simulink model "SPWM"  (R2018b)
settings: Solver=FixedStepAuto  StartTime=0.0  StopTime=0.02  RelTol=1e-3
undefined symbols (not defined in the file): gcbh, Newton, Raphson, sps_rtmsupport
libraries: powerlib x60, powerlib_meascontrol x21, simulink x14, dspstat3 x1
(part 1 of 2)
settings Model: Creator=Lenovo  LastModifiedBy=Lenovo

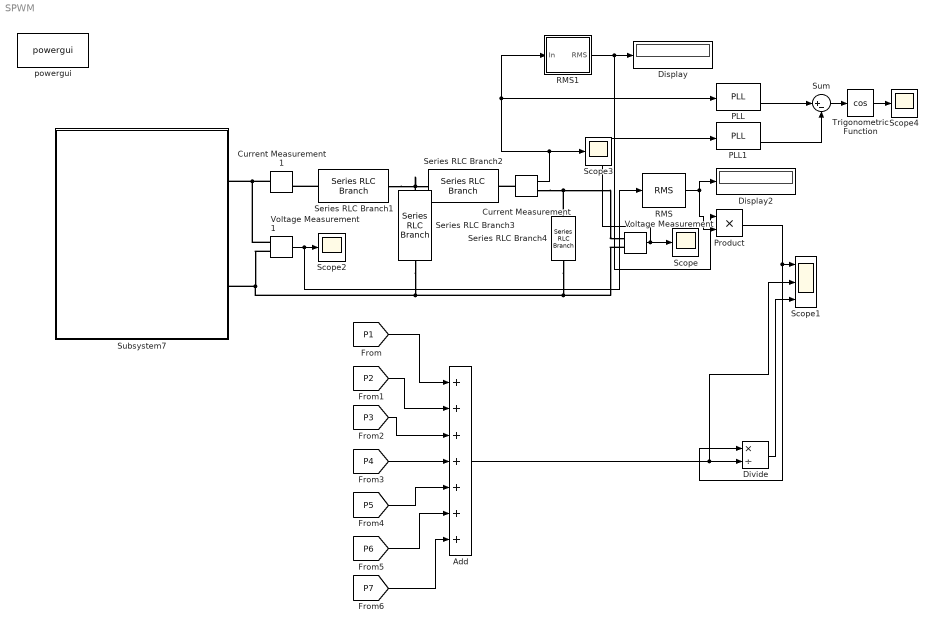
== system SPWM ==
  Add : Sum  Inputs=+++++++
  Current Measurement : powerlib/Measurements/Current Measurement  PhasorSimulation=off  OutputType=Complex  PSBequivalent=0
  Current Measurement1 : powerlib/Measurements/Current Measurement  PhasorSimulation=off  OutputType=Complex  PSBequivalent=0
  Display : Display
  Display2 : Display
  Divide : Product  Inputs=*/
  PLL : powerlib_meascontrol/PLL/PLL  Fmin=45  Par_Init=[0, 50]  ParK=[180, 3200, 1]  TcD=1e-4  MaxRateChangeFreq=12  FilterCutOffFreq=25  Ts=0  AGC=on
      settings: SourceProductName=Simscape Power Systems  SourceProductBaseCode=PS
  PLL1 : powerlib_meascontrol/PLL/PLL  Fmin=45  Par_Init=[0, 50]  ParK=[180, 3200, 1]  TcD=1e-4  MaxRateChangeFreq=12  FilterCutOffFreq=25  Ts=0  AGC=on
      settings: SourceProductName=Simscape Power Systems  SourceProductBaseCode=PS
  Product : Product
  RMS : powerlib_meascontrol/Measurements/RMS  TrueRMS=on  Freq=50  RMSInit=0  Ts=0
  RMS1 : Subsystem  DialogController=POWERSYS.PowerSysDialog  LoadFcn=sps_rtmsupport('LoadFcn', gcbh);  StartFcn=sps_rtmsupport('StartFcn', gcbh);  StopFcn=sps_rtmsupport('StopFcn', gcbh);  mask(RMS){TrueRMS=on, Freq=50, RMSInit=0, Ts=0}
      mask prompts: TrueRMS "True RMS value"; Freq "Fundamental frequency (Hz):"; RMSInit "Initial RMS value:"; Ts "Sample time:"
      mask help:
      | Measure the true root mean square (RMS) value of the input signal at the specified fundamental frequency.
      |
      | When True RMS value parameter is unchecked, the block outputs the RMS value of the fundamental component of the input signal.
      mask init:
      | [sps] = powericon('RMSInit',gcb,Freq,RMSInit,TrueRMS,Ts);
      settings: CopyFcn=sps_rtmsupport('CopyFcn', gcbh);  DeleteFcn=sps_rtmsupport('DeleteFcn', gcbh);  UndoDeleteFcn=sps_rtmsupport('UndoDeleteFcn', gcbh);  ModelCloseFcn=sps_rtmsupport('ModelCloseFcn', gcbh);  PreSaveFcn=sps_rtmsupport('PreSaveFcn', gcbh);  PostSaveFcn=sps_rtmsupport('PostSaveFcn', gcbh);  NameChangeFcn=sps_rtmsupport('NameChangeFcn', gcbh);  PreCopyFcn=sps_rtmsupport('PreCopyFcn', gcbh);  OpenFcn=sps_rtmsupport('OpenFcn', gcbh, [1]);  CloseFcn=sps_rtmsupport('CloseFcn', gcbh);  PreDeleteFcn=sps_rtmsupport('PreDeleteFcn', gcbh);
      mask Help: helpview(psbhelp);
      mask Display: color('blue');disp('RMS')
  Scope{,2..4} (4 alike) : Scope
  Scope1 : Scope  NumInputPorts=3
  Series RLC Branch1 : powerlib/Elements/Series RLC Branch  LConnTagsString=__new0  RConnTagsString=__new0  BranchType=L  Resistance=0.5  Inductance=0.32e-3  SetiL0=off  InitialCurrent=0  Capacitance=1e-6  Setx0=off  InitialVoltage=0  Measurements=None
  Series RLC Branch2 : powerlib/Elements/Series RLC Branch  LConnTagsString=__new0  RConnTagsString=__new0  BranchType=L  Resistance=0.5  Inductance=0.32e-3  SetiL0=off  InitialCurrent=0  Capacitance=1e-6  Setx0=off  InitialVoltage=0  Measurements=None
  Series RLC Branch3 : powerlib/Elements/Series RLC Branch  LConnTagsString=__new0  RConnTagsString=__new0  BranchType=C  Resistance=1  Inductance=1e-3  SetiL0=off  InitialCurrent=0  Capacitance=25e-4  Setx0=off  InitialVoltage=0  Measurements=None
  Series RLC Branch4 : powerlib/Elements/Series RLC Branch  LConnTagsString=__new0  RConnTagsString=__new0  BranchType=RL  Resistance=50  Inductance=50e-6  SetiL0=off  InitialCurrent=0  Capacitance=1e-6  Setx0=off  InitialVoltage=0  Measurements=None
  Subsystem7 : Subsystem
  Sum : Sum  Inputs=|+-
  Trigonometric Function : Trigonometry  Operator=cos
  Voltage Measurement : powerlib/Measurements/Voltage Measurement  PhasorSimulation=off  OutputType=Complex  PSBequivalent=0
  Voltage Measurement1 : powerlib/Measurements/Voltage Measurement  PhasorSimulation=off  OutputType=Complex  PSBequivalent=0
  powergui : powerlib/powergui  Priority=1  SimulationMode=Discrete  SampleTime=50e-6  frequency=60  Iterations=50  frequencyindice=0  Pbase=100e6  ErrMax=1e-4  UnitsV=kV  UnitsW=MW  buscounter=0  FunctionMessages=off  echomessages=off  EnableUseOfTLC=off  CurrentSourceSwitches=off  DisableSnubberDevices=off  DisableRonSwitches=off  DisableVfSwitches=off  DisplayEquations=off  SolverType=Tustin/Backward Euler (TBE)  Interpol=off  ExternalGateDelay=off  methode=off  Ts=100  x0status=blocks  SPID=off  SwTol=0  HookPort=off  RestoreLinks=warning  ResistiveCurrentMeasurement=off  Frange=[0:2:500]  Ylog=off  Xlog=on  ShowGrid=off  save=off  variable=ZData  structure=vinay3  ZoomFFT=off  StartTime=0.04  cycles=1  DisplayStyle=1  fundamental=50  FreqAxis=off  MaxFrequency=1000  frequencyindicesteady=1  RmsSteady=1  display=off
  wires:
  Voltage Measurement/1 -> PLL1/1, Scope/1
  Current Measurement/1 -> Scope3/1, RMS1/1(In), PLL/1
  Voltage Measurement1/1 -> RMS/1, Scope2/1
  RMS/1 -> Display2/1, Product/2
  [P1] -> Add/1
  [P2] -> Add/2
  [P3] -> Add/3
  [P4] -> Add/4
  [P5] -> Add/5
  [P6] -> Add/6
  [P7] -> Add/7
  Divide/1 -> Scope1/3
  RMS1/1(RMS) -> Product/1, Display/1
  Product/1 -> Divide/1, Scope1/1
  PLL/2 -> Sum/1
  PLL1/2 -> Sum/2
  Sum/1 -> Trigonometric Function/1
  Trigonometric Function/1 -> Scope4/1
  Add/1 -> Scope1/2, Divide/2
  connections:
  Subsystem7/RConn2 -- Series RLC Branch4/RConn1 -- Voltage Measurement/LConn2 -- Series RLC Branch3/RConn1 -- Voltage Measurement1/LConn2
  Series RLC Branch3/LConn1 -- Series RLC Branch1/RConn1 -- Series RLC Branch2/LConn1
  Voltage Measurement1/LConn1 -- Current Measurement1/LConn1 -- Subsystem7/RConn1
  Current Measurement/LConn1 -- Series RLC Branch2/RConn1
  Voltage Measurement/LConn1 -- Current Measurement/RConn1 -- Series RLC Branch4/LConn1
  Series RLC Branch1/LConn1 -- Current Measurement1/RConn1

== system SPWM/RMS1 ==
  In : Inport  SampleTime=Ts
  Constant : Constant  Value=TrueRMS
  Data Type Conversion : DataTypeConversion  OutDataTypeStr=boolean
  Logical Operator : Logic  Operator=NOT  AllPortsSameDT=off  OutDataTypeStr=boolean
  "RMS " : Subsystem
  Switch : Switch  Criteria=u2 ~= 0  Threshold=0.5
  "TrueRMS " : Subsystem
  RMS : Outport  SampleTime=Ts
  tag scope: Iooooobvw=global
  wires:
  In/1 -> "TrueRMS "/1(In), "RMS "/1(In)
  Switch/1 -> [Iooooobvw], RMS/1
  "TrueRMS "/1(RMS) -> Switch/1
  "RMS "/1(RMS) -> Switch/3
  Constant/1 -> Data Type Conversion/1
  Data Type Conversion/1 -> Logical Operator/1, "TrueRMS "/Enable, Switch/2
  Logical Operator/1 -> "RMS "/Enable

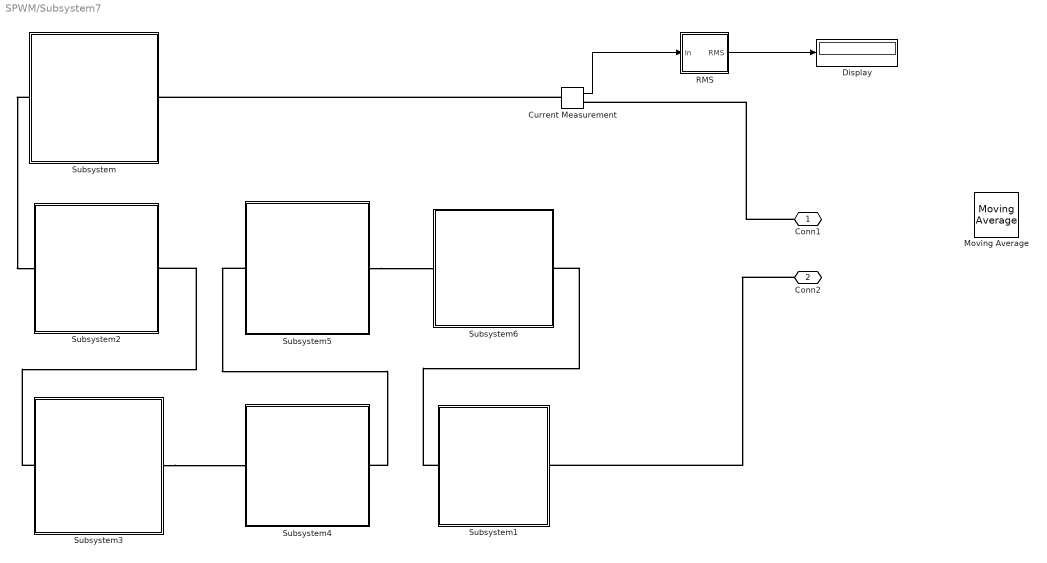
== system SPWM/Subsystem7 ==
  Current Measurement : powerlib/Measurements/Current Measurement  PhasorSimulation=off  OutputType=Complex  PSBequivalent=0
  Display : Display
  Moving Average : dspstat3/Moving Average  Method=Sliding window  ForgettingFactorPort=off  SpecifyWindowLength=on  WindowLength=4  ForgettingFactor=0.9  SimulateUsing=Code generation
  RMS : Subsystem  DialogController=POWERSYS.PowerSysDialog  LoadFcn=sps_rtmsupport('LoadFcn', gcbh);  StartFcn=sps_rtmsupport('StartFcn', gcbh);  StopFcn=sps_rtmsupport('StopFcn', gcbh);  mask(RMS){TrueRMS=on, Freq=50, RMSInit=0, Ts=0}
      mask prompts: TrueRMS "True RMS value"; Freq "Fundamental frequency (Hz):"; RMSInit "Initial RMS value:"; Ts "Sample time:"
      mask help:
      | Measure the true root mean square (RMS) value of the input signal at the specified fundamental frequency.
      |
      | When True RMS value parameter is unchecked, the block outputs the RMS value of the fundamental component of the input signal.
      mask init:
      | [sps] = powericon('RMSInit',gcb,Freq,RMSInit,TrueRMS,Ts);
      settings: CopyFcn=sps_rtmsupport('CopyFcn', gcbh);  DeleteFcn=sps_rtmsupport('DeleteFcn', gcbh);  UndoDeleteFcn=sps_rtmsupport('UndoDeleteFcn', gcbh);  ModelCloseFcn=sps_rtmsupport('ModelCloseFcn', gcbh);  PreSaveFcn=sps_rtmsupport('PreSaveFcn', gcbh);  PostSaveFcn=sps_rtmsupport('PostSaveFcn', gcbh);  NameChangeFcn=sps_rtmsupport('NameChangeFcn', gcbh);  PreCopyFcn=sps_rtmsupport('PreCopyFcn', gcbh);  OpenFcn=sps_rtmsupport('OpenFcn', gcbh, [1]);  CloseFcn=sps_rtmsupport('CloseFcn', gcbh);  PreDeleteFcn=sps_rtmsupport('PreDeleteFcn', gcbh);
      mask Help: helpview(psbhelp);
      mask Display: color('blue');disp('RMS')
  Subsystem : Subsystem
  Subsystem1 : Subsystem
  Subsystem2 : Subsystem
  Subsystem3 : Subsystem
  Subsystem4 : Subsystem
  Subsystem5 : Subsystem
  Subsystem6 : Subsystem
  Conn1 : PMIOPort  Side=Right
  Conn2 : PMIOPort  Port=2  Side=Right
  wires:
  Current Measurement/1 -> RMS/1(In)
  RMS/1(RMS) -> Display/1
  connections:
  Conn2/RConn1 -- Subsystem1/RConn1
  Subsystem5/LConn1 -- Subsystem4/RConn1
  Subsystem3/RConn1 -- Subsystem4/LConn1
  Subsystem1/LConn1 -- Subsystem6/RConn1
  Subsystem5/RConn1 -- Subsystem6/LConn1
  Subsystem3/LConn1 -- Subsystem2/RConn1
  Current Measurement/LConn1 -- Subsystem/RConn1
  Subsystem/LConn1 -- Subsystem2/LConn1
  Conn1/RConn1 -- Current Measurement/RConn1

== system SPWM/RMS1/RMS  ==
  In : Inport
  Enable : EnablePort
  Fourier1 : powerlib_meascontrol/Measurements/Fourier  Freq=sps.Freq  n=1  InInit=sps.Par_Init_RMS  Ts=Ts
      settings: SourceProductName=Simscape Power Systems
  Gain : Gain  Gain=1/sqrt(2)
  Terminator : Terminator
  RMS : Outport
  wires:
  Fourier1/1 -> Gain/1
  Fourier1/2 -> Terminator/1
  In/1 -> Fourier1/1
  Gain/1 -> RMS/1

== system SPWM/RMS1/TrueRMS  ==
  In : Inport
  Enable : EnablePort
  Mean value : powerlib_meascontrol/Measurements/Mean  Freq=sps.Freq  Vinit=sps.Par_Init_TrueRMS  Ts=Ts
  Product : Product  SaturateOnIntegerOverflow=on  InputSameDT=on  OutDataTypeStr=Inherit: Same as first input
  Saturation to avoid negative sqrt : Saturate  UpperLimit=Inf  LowerLimit=0
  Sqrt : Sqrt  AlgorithmType=Newton-Raphson  SaturateOnIntegerOverflow=on
  RMS : Outport
  wires:
  Saturation to avoid negative sqrt/1 -> Sqrt/1
  Mean value/1 -> Saturation to avoid negative sqrt/1
  Product/1 -> Mean value/1
  In/1 -> Product/2, Product/1
  Sqrt/1 -> RMS/1

== system SPWM/Subsystem7/RMS ==
  In : Inport  SampleTime=Ts
  Constant : Constant  Value=TrueRMS
  Data Type Conversion : DataTypeConversion  OutDataTypeStr=boolean
  Logical Operator : Logic  Operator=NOT  AllPortsSameDT=off  OutDataTypeStr=boolean
  "RMS " : Subsystem
  Subsystem : Subsystem
  Switch : Switch  Criteria=u2 ~= 0  Threshold=0.5
  "TrueRMS " : Subsystem
  RMS : Outport  SampleTime=Ts
  wires:
  In/1 -> "TrueRMS "/1(In), "RMS "/1(In)
  "TrueRMS "/1(RMS) -> Switch/1
  "RMS "/1(RMS) -> Switch/3
  Constant/1 -> Data Type Conversion/1
  Data Type Conversion/1 -> Logical Operator/1, "TrueRMS "/Enable, Switch/2
  Logical Operator/1 -> "RMS "/Enable
  Switch/1 -> Subsystem/1(In1)
  Subsystem/1(Out1) -> RMS/1

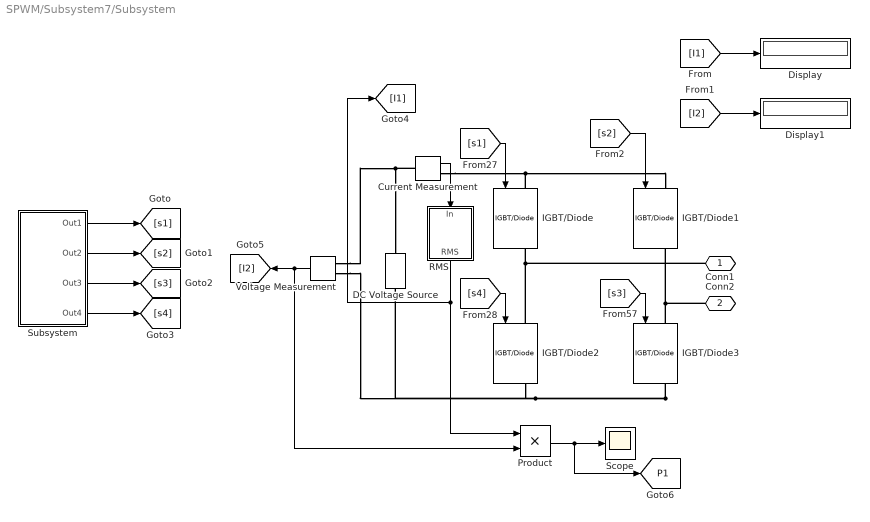
== system SPWM/Subsystem7/Subsystem ==
  Current Measurement : powerlib/Measurements/Current Measurement  PhasorSimulation=off  OutputType=Complex  PSBequivalent=0
  DC Voltage Source : powerlib/Electrical Sources/DC Voltage Source  Amplitude=46.42  Measurements=None
  Display : Display
      settings: Decimation=2
  Display1 : Display
  IGBT/Diode{,1..3} (4 alike) : powerlib/Power Electronics/IGBT//Diode  Ron=0.002  Rs=1e5  Cs=inf  Measurements=on
  Product : Product
  RMS : Subsystem  DialogController=POWERSYS.PowerSysDialog  LoadFcn=sps_rtmsupport('LoadFcn', gcbh);  StartFcn=sps_rtmsupport('StartFcn', gcbh);  StopFcn=sps_rtmsupport('StopFcn', gcbh);  mask(RMS){TrueRMS=on, Freq=50, RMSInit=0, Ts=0}
      mask prompts: TrueRMS "True RMS value"; Freq "Fundamental frequency (Hz):"; RMSInit "Initial RMS value:"; Ts "Sample time:"
      mask help:
      | Measure the true root mean square (RMS) value of the input signal at the specified fundamental frequency.
      |
      | When True RMS value parameter is unchecked, the block outputs the RMS value of the fundamental component of the input signal.
      mask init:
      | [sps] = powericon('RMSInit',gcb,Freq,RMSInit,TrueRMS,Ts);
      settings: CopyFcn=sps_rtmsupport('CopyFcn', gcbh);  DeleteFcn=sps_rtmsupport('DeleteFcn', gcbh);  UndoDeleteFcn=sps_rtmsupport('UndoDeleteFcn', gcbh);  ModelCloseFcn=sps_rtmsupport('ModelCloseFcn', gcbh);  PreSaveFcn=sps_rtmsupport('PreSaveFcn', gcbh);  PostSaveFcn=sps_rtmsupport('PostSaveFcn', gcbh);  NameChangeFcn=sps_rtmsupport('NameChangeFcn', gcbh);  PreCopyFcn=sps_rtmsupport('PreCopyFcn', gcbh);  OpenFcn=sps_rtmsupport('OpenFcn', gcbh, [1]);  CloseFcn=sps_rtmsupport('CloseFcn', gcbh);  PreDeleteFcn=sps_rtmsupport('PreDeleteFcn', gcbh);
      mask Help: helpview(psbhelp);
      mask Display: color('blue');disp('RMS')
  Scope : Scope
  Subsystem : Subsystem
  Voltage Measurement : powerlib/Measurements/Voltage Measurement  PhasorSimulation=off  OutputType=Complex  PSBequivalent=0
  Conn1 : PMIOPort  Side=Right
  Conn2 : PMIOPort  Port=2  Side=Left
  tag scope: P1=global
  wires:
  [s1] -> IGBT/Diode/1
  [s4] -> IGBT/Diode2/1
  [s3] -> IGBT/Diode3/1
  [s2] -> IGBT/Diode1/1
  Subsystem/1(Out1) -> [s1]
  Subsystem/2(Out2) -> [s2]
  Subsystem/3(Out3) -> [s3]
  Subsystem/4(Out4) -> [s4]
  Voltage Measurement/1 -> Product/2, [I2]
  [I1] -> Display/1
  Current Measurement/1 -> RMS/1(In)
  [I2] -> Display1/1
  Product/1 -> [P1], Scope/1
  RMS/1(RMS) -> [I1], Product/1
  connections:
  IGBT/Diode3/RConn1 -- IGBT/Diode2/RConn1 -- DC Voltage Source/LConn1 -- Voltage Measurement/LConn2
  IGBT/Diode/LConn1 -- IGBT/Diode1/LConn1 -- Current Measurement/RConn1
  IGBT/Diode3/LConn1 -- Conn2/RConn1 -- IGBT/Diode1/RConn1
  IGBT/Diode/RConn1 -- IGBT/Diode2/LConn1 -- Conn1/RConn1
  Current Measurement/LConn1 -- DC Voltage Source/RConn1 -- Voltage Measurement/LConn1

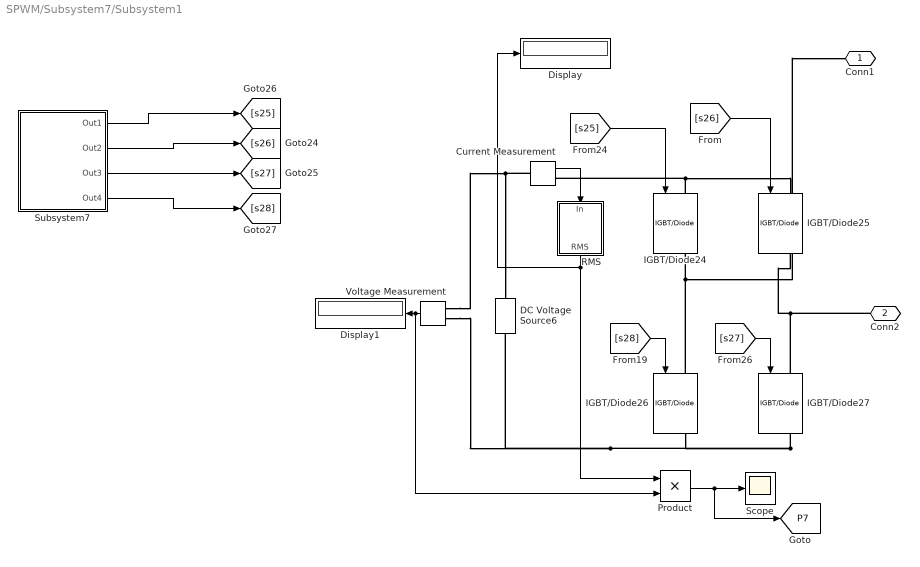
== system SPWM/Subsystem7/Subsystem1 ==
  Current Measurement : powerlib/Measurements/Current Measurement  PhasorSimulation=off  OutputType=Complex  PSBequivalent=0
  DC Voltage Source6 : powerlib/Electrical Sources/DC Voltage Source  Amplitude=46.42  Measurements=None
  Display : Display
  Display1 : Display
  IGBT/Diode{24..27} (4 alike) : powerlib/Power Electronics/IGBT//Diode  Ron=0.002  Rs=1e5  Cs=inf  Measurements=on
  Product : Product
  RMS : Subsystem  DialogController=POWERSYS.PowerSysDialog  LoadFcn=sps_rtmsupport('LoadFcn', gcbh);  StartFcn=sps_rtmsupport('StartFcn', gcbh);  StopFcn=sps_rtmsupport('StopFcn', gcbh);  mask(RMS){TrueRMS=on, Freq=50, RMSInit=0, Ts=0}
      mask prompts: TrueRMS "True RMS value"; Freq "Fundamental frequency (Hz):"; RMSInit "Initial RMS value:"; Ts "Sample time:"
      mask help:
      | Measure the true root mean square (RMS) value of the input signal at the specified fundamental frequency.
      |
      | When True RMS value parameter is unchecked, the block outputs the RMS value of the fundamental component of the input signal.
      mask init:
      | [sps] = powericon('RMSInit',gcb,Freq,RMSInit,TrueRMS,Ts);
      settings: CopyFcn=sps_rtmsupport('CopyFcn', gcbh);  DeleteFcn=sps_rtmsupport('DeleteFcn', gcbh);  UndoDeleteFcn=sps_rtmsupport('UndoDeleteFcn', gcbh);  ModelCloseFcn=sps_rtmsupport('ModelCloseFcn', gcbh);  PreSaveFcn=sps_rtmsupport('PreSaveFcn', gcbh);  PostSaveFcn=sps_rtmsupport('PostSaveFcn', gcbh);  NameChangeFcn=sps_rtmsupport('NameChangeFcn', gcbh);  PreCopyFcn=sps_rtmsupport('PreCopyFcn', gcbh);  OpenFcn=sps_rtmsupport('OpenFcn', gcbh, [1]);  CloseFcn=sps_rtmsupport('CloseFcn', gcbh);  PreDeleteFcn=sps_rtmsupport('PreDeleteFcn', gcbh);
      mask Help: helpview(psbhelp);
      mask Display: color('blue');disp('RMS')
  Scope : Scope
  Subsystem7 : Subsystem
  Voltage Measurement : powerlib/Measurements/Voltage Measurement  PhasorSimulation=off  OutputType=Complex  PSBequivalent=0
  Conn1 : PMIOPort  Side=Left
  Conn2 : PMIOPort  Port=2  Side=Right
  tag scope: P7=global
  wires:
  [s27] -> IGBT/Diode27/1
  [s28] -> IGBT/Diode26/1
  [s25] -> IGBT/Diode24/1
  Subsystem7/4(Out4) -> [s28]
  Subsystem7/3(Out3) -> [s27]
  Subsystem7/1(Out1) -> [s25]
  Subsystem7/2(Out2) -> [s26]
  [s26] -> IGBT/Diode25/1
  Voltage Measurement/1 -> Product/2, Display1/1
  Current Measurement/1 -> RMS/1(In)
  Product/1 -> [P7], Scope/1
  RMS/1(RMS) -> Product/1, Display/1
  connections:
  IGBT/Diode27/RConn1 -- IGBT/Diode26/RConn1 -- DC Voltage Source6/LConn1 -- Voltage Measurement/LConn2
  Current Measurement/LConn1 -- DC Voltage Source6/RConn1 -- Voltage Measurement/LConn1
  IGBT/Diode27/LConn1 -- IGBT/Diode25/RConn1 -- Conn2/RConn1
  IGBT/Diode26/LConn1 -- IGBT/Diode24/RConn1 -- Conn1/RConn1
  IGBT/Diode24/LConn1 -- Current Measurement/RConn1 -- IGBT/Diode25/LConn1

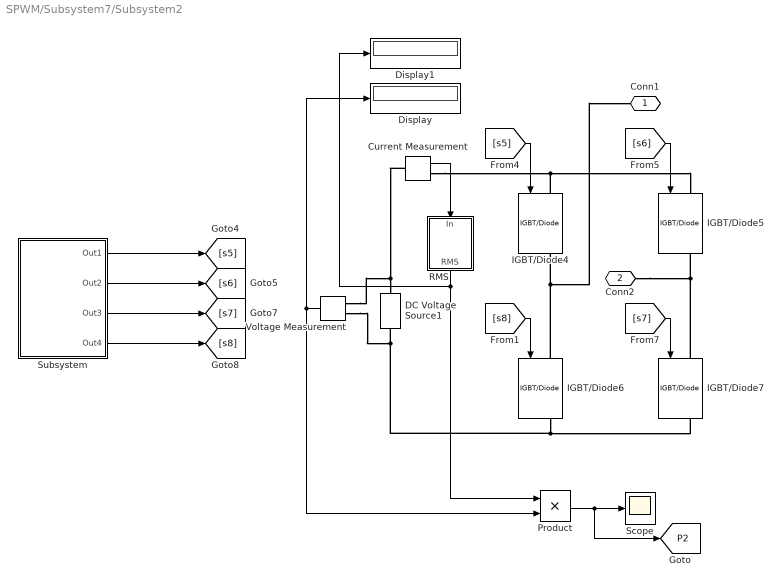
== system SPWM/Subsystem7/Subsystem2 ==
  Current Measurement : powerlib/Measurements/Current Measurement  PhasorSimulation=off  OutputType=Complex  PSBequivalent=0
  DC Voltage Source1 : powerlib/Electrical Sources/DC Voltage Source  Amplitude=46.42  Measurements=None
  Display : Display
  Display1 : Display
  IGBT/Diode{4..7} (4 alike) : powerlib/Power Electronics/IGBT//Diode  Ron=0.002  Rs=1e5  Cs=inf  Measurements=on
  Product : Product
  RMS : Subsystem  DialogController=POWERSYS.PowerSysDialog  LoadFcn=sps_rtmsupport('LoadFcn', gcbh);  StartFcn=sps_rtmsupport('StartFcn', gcbh);  StopFcn=sps_rtmsupport('StopFcn', gcbh);  mask(RMS){TrueRMS=on, Freq=50, RMSInit=0, Ts=0}
      mask prompts: TrueRMS "True RMS value"; Freq "Fundamental frequency (Hz):"; RMSInit "Initial RMS value:"; Ts "Sample time:"
      mask help:
      | Measure the true root mean square (RMS) value of the input signal at the specified fundamental frequency.
      |
      | When True RMS value parameter is unchecked, the block outputs the RMS value of the fundamental component of the input signal.
      mask init:
      | [sps] = powericon('RMSInit',gcb,Freq,RMSInit,TrueRMS,Ts);
      settings: CopyFcn=sps_rtmsupport('CopyFcn', gcbh);  DeleteFcn=sps_rtmsupport('DeleteFcn', gcbh);  UndoDeleteFcn=sps_rtmsupport('UndoDeleteFcn', gcbh);  ModelCloseFcn=sps_rtmsupport('ModelCloseFcn', gcbh);  PreSaveFcn=sps_rtmsupport('PreSaveFcn', gcbh);  PostSaveFcn=sps_rtmsupport('PostSaveFcn', gcbh);  NameChangeFcn=sps_rtmsupport('NameChangeFcn', gcbh);  PreCopyFcn=sps_rtmsupport('PreCopyFcn', gcbh);  OpenFcn=sps_rtmsupport('OpenFcn', gcbh, [1]);  CloseFcn=sps_rtmsupport('CloseFcn', gcbh);  PreDeleteFcn=sps_rtmsupport('PreDeleteFcn', gcbh);
      mask Help: helpview(psbhelp);
      mask Display: color('blue');disp('RMS')
  Scope : Scope
  Subsystem : Subsystem
  Voltage Measurement : powerlib/Measurements/Voltage Measurement  PhasorSimulation=off  OutputType=Complex  PSBequivalent=0
  Conn1 : PMIOPort  Side=Left
  Conn2 : PMIOPort  Port=2  Side=Right
  tag scope: P2=global
  wires:
  [s8] -> IGBT/Diode6/1
  [s6] -> IGBT/Diode5/1
  [s5] -> IGBT/Diode4/1
  [s7] -> IGBT/Diode7/1
  Subsystem/1(Out1) -> [s5]
  Subsystem/2(Out2) -> [s6]
  Subsystem/3(Out3) -> [s7]
  Subsystem/4(Out4) -> [s8]
  Voltage Measurement/1 -> Display/1, Product/2
  Current Measurement/1 -> RMS/1(In)
  Product/1 -> [P2], Scope/1
  RMS/1(RMS) -> Product/1, Display1/1
  connections:
  IGBT/Diode7/LConn1 -- Conn2/RConn1 -- IGBT/Diode5/RConn1
  DC Voltage Source1/RConn1 -- Current Measurement/LConn1 -- Voltage Measurement/LConn1
  IGBT/Diode6/LConn1 -- IGBT/Diode4/RConn1 -- Conn1/RConn1
  IGBT/Diode7/RConn1 -- IGBT/Diode6/RConn1 -- Voltage Measurement/LConn2 -- DC Voltage Source1/LConn1
  Current Measurement/RConn1 -- IGBT/Diode4/LConn1 -- IGBT/Diode5/LConn1

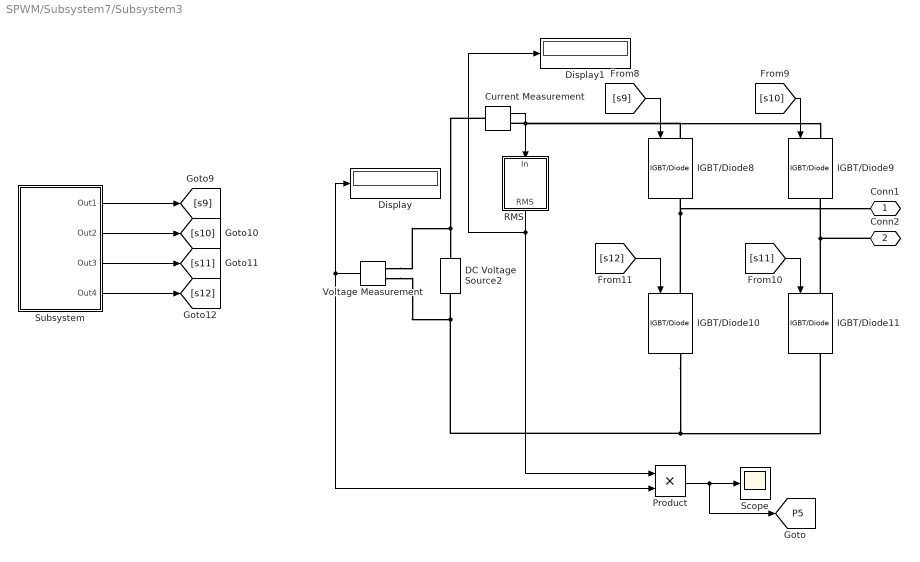
== system SPWM/Subsystem7/Subsystem3 ==
  Current Measurement : powerlib/Measurements/Current Measurement  PhasorSimulation=off  OutputType=Complex  PSBequivalent=0
  DC Voltage Source2 : powerlib/Electrical Sources/DC Voltage Source  Amplitude=46.42  Measurements=None
  Display : Display
  Display1 : Display
  IGBT/Diode{8..11} (4 alike) : powerlib/Power Electronics/IGBT//Diode  Ron=0.002  Rs=1e5  Cs=inf  Measurements=on
  Product : Product
  RMS : Subsystem  DialogController=POWERSYS.PowerSysDialog  LoadFcn=sps_rtmsupport('LoadFcn', gcbh);  StartFcn=sps_rtmsupport('StartFcn', gcbh);  StopFcn=sps_rtmsupport('StopFcn', gcbh);  mask(RMS){TrueRMS=on, Freq=50, RMSInit=0, Ts=0}
      mask prompts: TrueRMS "True RMS value"; Freq "Fundamental frequency (Hz):"; RMSInit "Initial RMS value:"; Ts "Sample time:"
      mask help:
      | Measure the true root mean square (RMS) value of the input signal at the specified fundamental frequency.
      |
      | When True RMS value parameter is unchecked, the block outputs the RMS value of the fundamental component of the input signal.
      mask init:
      | [sps] = powericon('RMSInit',gcb,Freq,RMSInit,TrueRMS,Ts);
      settings: CopyFcn=sps_rtmsupport('CopyFcn', gcbh);  DeleteFcn=sps_rtmsupport('DeleteFcn', gcbh);  UndoDeleteFcn=sps_rtmsupport('UndoDeleteFcn', gcbh);  ModelCloseFcn=sps_rtmsupport('ModelCloseFcn', gcbh);  PreSaveFcn=sps_rtmsupport('PreSaveFcn', gcbh);  PostSaveFcn=sps_rtmsupport('PostSaveFcn', gcbh);  NameChangeFcn=sps_rtmsupport('NameChangeFcn', gcbh);  PreCopyFcn=sps_rtmsupport('PreCopyFcn', gcbh);  OpenFcn=sps_rtmsupport('OpenFcn', gcbh, [1]);  CloseFcn=sps_rtmsupport('CloseFcn', gcbh);  PreDeleteFcn=sps_rtmsupport('PreDeleteFcn', gcbh);
      mask Help: helpview(psbhelp);
      mask Display: color('blue');disp('RMS')
  Scope : Scope
  Subsystem : Subsystem
  Voltage Measurement : powerlib/Measurements/Voltage Measurement  PhasorSimulation=off  OutputType=Complex  PSBequivalent=0
  Conn1 : PMIOPort  Side=Left
  Conn2 : PMIOPort  Port=2  Side=Right
  tag scope: P5=global
  wires:
  [s11] -> IGBT/Diode11/1
  [s9] -> IGBT/Diode8/1
  [s10] -> IGBT/Diode9/1
  [s12] -> IGBT/Diode10/1
  Subsystem/1(Out1) -> [s9]
  Subsystem/2(Out2) -> [s10]
  Subsystem/3(Out3) -> [s11]
  Subsystem/4(Out4) -> [s12]
  Current Measurement/1 -> RMS/1(In)
  Voltage Measurement/1 -> Display/1, Product/2
  Product/1 -> [P5], Scope/1
  RMS/1(RMS) -> Product/1, Display1/1
  connections:
  Current Measurement/RConn1 -- IGBT/Diode9/LConn1 -- IGBT/Diode8/LConn1
  IGBT/Diode10/LConn1 -- IGBT/Diode8/RConn1 -- Conn1/RConn1
  Conn2/RConn1 -- IGBT/Diode11/LConn1 -- IGBT/Diode9/RConn1
  IGBT/Diode10/RConn1 -- IGBT/Diode11/RConn1 -- DC Voltage Source2/LConn1 -- Voltage Measurement/LConn2
  Current Measurement/LConn1 -- DC Voltage Source2/RConn1 -- Voltage Measurement/LConn1

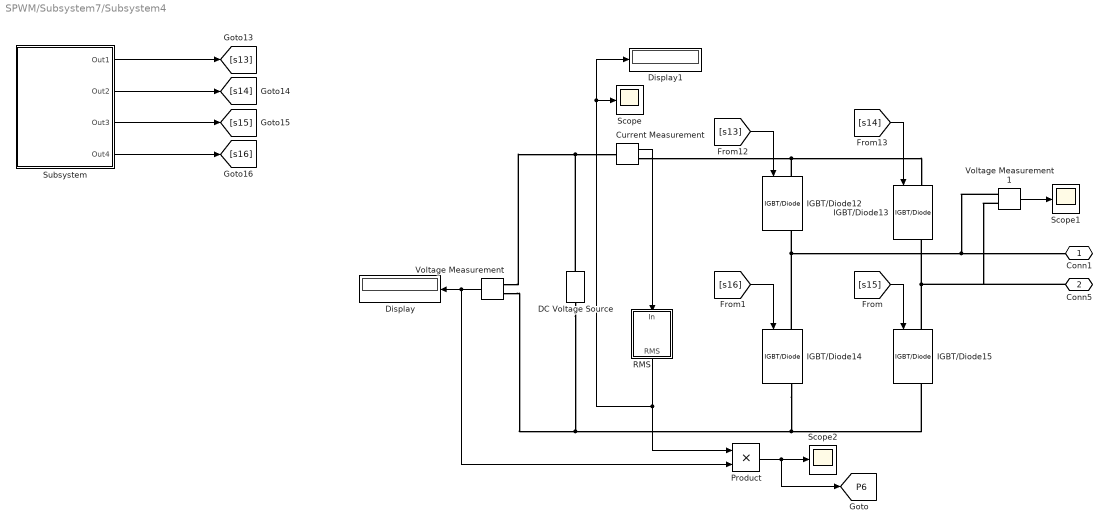
== system SPWM/Subsystem7/Subsystem4 ==
  Current Measurement : powerlib/Measurements/Current Measurement  PhasorSimulation=off  OutputType=Complex  PSBequivalent=0
  DC Voltage Source : powerlib/Electrical Sources/DC Voltage Source  Amplitude=46.42  Measurements=None
  Display : Display
  Display1 : Display
  IGBT/Diode{12..15} (4 alike) : powerlib/Power Electronics/IGBT//Diode  Ron=0.002  Rs=1e5  Cs=inf  Measurements=on
  Product : Product
  RMS : Subsystem  DialogController=POWERSYS.PowerSysDialog  LoadFcn=sps_rtmsupport('LoadFcn', gcbh);  StartFcn=sps_rtmsupport('StartFcn', gcbh);  StopFcn=sps_rtmsupport('StopFcn', gcbh);  mask(RMS){TrueRMS=on, Freq=50, RMSInit=0, Ts=0}
      mask prompts: TrueRMS "True RMS value"; Freq "Fundamental frequency (Hz):"; RMSInit "Initial RMS value:"; Ts "Sample time:"
      mask help:
      | Measure the true root mean square (RMS) value of the input signal at the specified fundamental frequency.
      |
      | When True RMS value parameter is unchecked, the block outputs the RMS value of the fundamental component of the input signal.
      mask init:
      | [sps] = powericon('RMSInit',gcb,Freq,RMSInit,TrueRMS,Ts);
      settings: CopyFcn=sps_rtmsupport('CopyFcn', gcbh);  DeleteFcn=sps_rtmsupport('DeleteFcn', gcbh);  UndoDeleteFcn=sps_rtmsupport('UndoDeleteFcn', gcbh);  ModelCloseFcn=sps_rtmsupport('ModelCloseFcn', gcbh);  PreSaveFcn=sps_rtmsupport('PreSaveFcn', gcbh);  PostSaveFcn=sps_rtmsupport('PostSaveFcn', gcbh);  NameChangeFcn=sps_rtmsupport('NameChangeFcn', gcbh);  PreCopyFcn=sps_rtmsupport('PreCopyFcn', gcbh);  OpenFcn=sps_rtmsupport('OpenFcn', gcbh, [1]);  CloseFcn=sps_rtmsupport('CloseFcn', gcbh);  PreDeleteFcn=sps_rtmsupport('PreDeleteFcn', gcbh);
      mask Help: helpview(psbhelp);
      mask Display: color('blue');disp('RMS')
  Scope : Scope
  Scope1 : Scope
  Scope2 : Scope
  Subsystem : Subsystem
  Voltage Measurement : powerlib/Measurements/Voltage Measurement  PhasorSimulation=off  OutputType=Complex  PSBequivalent=0
  Voltage Measurement1 : powerlib/Measurements/Voltage Measurement  PhasorSimulation=off  OutputType=Complex  PSBequivalent=0
  Conn1 : PMIOPort  Side=Left
  Conn5 : PMIOPort  Port=2  Side=Right
  tag scope: P6=global
  wires:
  [s14] -> IGBT/Diode13/1
  [s15] -> IGBT/Diode15/1
  [s16] -> IGBT/Diode14/1
  [s13] -> IGBT/Diode12/1
  Subsystem/1(Out1) -> [s13]
  Subsystem/2(Out2) -> [s14]
  Subsystem/3(Out3) -> [s15]
  Subsystem/4(Out4) -> [s16]
  Voltage Measurement/1 -> Product/2, Display/1
  Current Measurement/1 -> RMS/1(In)
  Voltage Measurement1/1 -> Scope1/1
  Product/1 -> [P6], Scope2/1
  RMS/1(RMS) -> Display1/1, Scope/1, Product/1
  connections:
  IGBT/Diode14/LConn1 -- IGBT/Diode12/RConn1 -- Voltage Measurement1/LConn1 -- Conn1/RConn1
  IGBT/Diode15/LConn1 -- Voltage Measurement1/LConn2 -- Conn5/RConn1 -- IGBT/Diode13/RConn1
  Voltage Measurement/LConn1 -- DC Voltage Source/RConn1 -- Current Measurement/LConn1
  IGBT/Diode12/LConn1 -- Current Measurement/RConn1 -- IGBT/Diode13/LConn1
  Voltage Measurement/LConn2 -- DC Voltage Source/LConn1 -- IGBT/Diode14/RConn1 -- IGBT/Diode15/RConn1

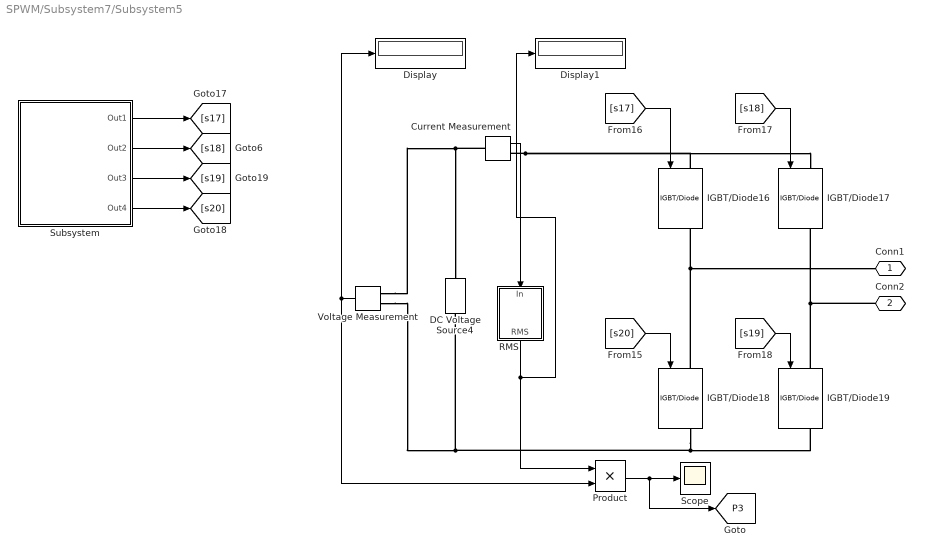
== system SPWM/Subsystem7/Subsystem5 ==
  Current Measurement : powerlib/Measurements/Current Measurement  PhasorSimulation=off  OutputType=Complex  PSBequivalent=0
  DC Voltage Source4 : powerlib/Electrical Sources/DC Voltage Source  Amplitude=46.42  Measurements=None
  Display : Display
  Display1 : Display
  IGBT/Diode{16..19} (4 alike) : powerlib/Power Electronics/IGBT//Diode  Ron=0.002  Rs=1e5  Cs=inf  Measurements=on
  Product : Product
  RMS : Subsystem  DialogController=POWERSYS.PowerSysDialog  LoadFcn=sps_rtmsupport('LoadFcn', gcbh);  StartFcn=sps_rtmsupport('StartFcn', gcbh);  StopFcn=sps_rtmsupport('StopFcn', gcbh);  mask(RMS){TrueRMS=on, Freq=50, RMSInit=0, Ts=0}
      mask prompts: TrueRMS "True RMS value"; Freq "Fundamental frequency (Hz):"; RMSInit "Initial RMS value:"; Ts "Sample time:"
      mask help:
      | Measure the true root mean square (RMS) value of the input signal at the specified fundamental frequency.
      |
      | When True RMS value parameter is unchecked, the block outputs the RMS value of the fundamental component of the input signal.
      mask init:
      | [sps] = powericon('RMSInit',gcb,Freq,RMSInit,TrueRMS,Ts);
      settings: CopyFcn=sps_rtmsupport('CopyFcn', gcbh);  DeleteFcn=sps_rtmsupport('DeleteFcn', gcbh);  UndoDeleteFcn=sps_rtmsupport('UndoDeleteFcn', gcbh);  ModelCloseFcn=sps_rtmsupport('ModelCloseFcn', gcbh);  PreSaveFcn=sps_rtmsupport('PreSaveFcn', gcbh);  PostSaveFcn=sps_rtmsupport('PostSaveFcn', gcbh);  NameChangeFcn=sps_rtmsupport('NameChangeFcn', gcbh);  PreCopyFcn=sps_rtmsupport('PreCopyFcn', gcbh);  OpenFcn=sps_rtmsupport('OpenFcn', gcbh, [1]);  CloseFcn=sps_rtmsupport('CloseFcn', gcbh);  PreDeleteFcn=sps_rtmsupport('PreDeleteFcn', gcbh);
      mask Help: helpview(psbhelp);
      mask Display: color('blue');disp('RMS')
  Scope : Scope
  Subsystem : Subsystem
  Voltage Measurement : powerlib/Measurements/Voltage Measurement  PhasorSimulation=off  OutputType=Complex  PSBequivalent=0
  Conn1 : PMIOPort  Side=Left
  Conn2 : PMIOPort  Port=2  Side=Right
  tag scope: P3=global
  wires:
  [s18] -> IGBT/Diode17/1
  [s17] -> IGBT/Diode16/1
  [s19] -> IGBT/Diode19/1
  [s20] -> IGBT/Diode18/1
  Subsystem/1(Out1) -> [s17]
  Subsystem/2(Out2) -> [s18]
  Subsystem/3(Out3) -> [s19]
  Subsystem/4(Out4) -> [s20]
  Voltage Measurement/1 -> Display/1, Product/2
  Current Measurement/1 -> RMS/1(In)
  Product/1 -> [P3], Scope/1
  RMS/1(RMS) -> Display1/1, Product/1
  connections:
  IGBT/Diode18/RConn1 -- Voltage Measurement/LConn2 -- DC Voltage Source4/LConn1 -- IGBT/Diode19/RConn1
  IGBT/Diode18/LConn1 -- IGBT/Diode16/RConn1 -- Conn1/RConn1
  Current Measurement/RConn1 -- IGBT/Diode17/LConn1 -- IGBT/Diode16/LConn1
  IGBT/Diode19/LConn1 -- IGBT/Diode17/RConn1 -- Conn2/RConn1
  Voltage Measurement/LConn1 -- Current Measurement/LConn1 -- DC Voltage Source4/RConn1

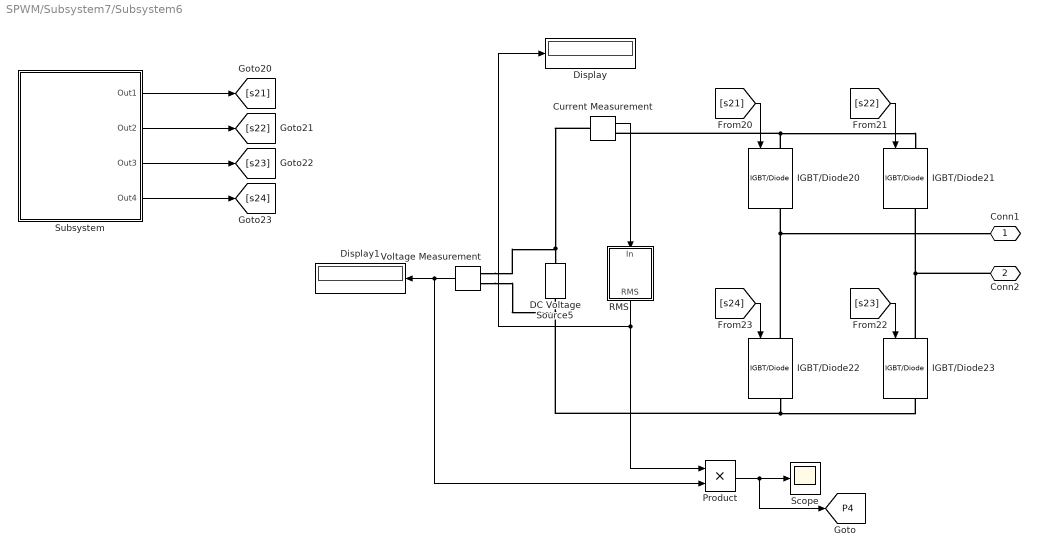
== system SPWM/Subsystem7/Subsystem6 ==
  Current Measurement : powerlib/Measurements/Current Measurement  PhasorSimulation=off  OutputType=Complex  PSBequivalent=0
  DC Voltage Source5 : powerlib/Electrical Sources/DC Voltage Source  Amplitude=46.42  Measurements=None
  Display : Display
  Display1 : Display
  IGBT/Diode{20..23} (4 alike) : powerlib/Power Electronics/IGBT//Diode  Ron=0.002  Rs=1e5  Cs=inf  Measurements=on
  Product : Product
  RMS : Subsystem  DialogController=POWERSYS.PowerSysDialog  LoadFcn=sps_rtmsupport('LoadFcn', gcbh);  StartFcn=sps_rtmsupport('StartFcn', gcbh);  StopFcn=sps_rtmsupport('StopFcn', gcbh);  mask(RMS){TrueRMS=on, Freq=50, RMSInit=0, Ts=0}
      mask prompts: TrueRMS "True RMS value"; Freq "Fundamental frequency (Hz):"; RMSInit "Initial RMS value:"; Ts "Sample time:"
      mask help:
      | Measure the true root mean square (RMS) value of the input signal at the specified fundamental frequency.
      |
      | When True RMS value parameter is unchecked, the block outputs the RMS value of the fundamental component of the input signal.
      mask init:
      | [sps] = powericon('RMSInit',gcb,Freq,RMSInit,TrueRMS,Ts);
      settings: CopyFcn=sps_rtmsupport('CopyFcn', gcbh);  DeleteFcn=sps_rtmsupport('DeleteFcn', gcbh);  UndoDeleteFcn=sps_rtmsupport('UndoDeleteFcn', gcbh);  ModelCloseFcn=sps_rtmsupport('ModelCloseFcn', gcbh);  PreSaveFcn=sps_rtmsupport('PreSaveFcn', gcbh);  PostSaveFcn=sps_rtmsupport('PostSaveFcn', gcbh);  NameChangeFcn=sps_rtmsupport('NameChangeFcn', gcbh);  PreCopyFcn=sps_rtmsupport('PreCopyFcn', gcbh);  OpenFcn=sps_rtmsupport('OpenFcn', gcbh, [1]);  CloseFcn=sps_rtmsupport('CloseFcn', gcbh);  PreDeleteFcn=sps_rtmsupport('PreDeleteFcn', gcbh);
      mask Help: helpview(psbhelp);
      mask Display: color('blue');disp('RMS')
  Scope : Scope
  Subsystem : Subsystem
  Voltage Measurement : powerlib/Measurements/Voltage Measurement  PhasorSimulation=off  OutputType=Complex  PSBequivalent=0
  Conn1 : PMIOPort  Side=Left
  Conn2 : PMIOPort  Port=2  Side=Right
  tag scope: P4=global
  wires:
  [s22] -> IGBT/Diode21/1
  [s23] -> IGBT/Diode23/1
  [s21] -> IGBT/Diode20/1
  [s24] -> IGBT/Diode22/1
  Subsystem/1(Out1) -> [s21]
  Subsystem/2(Out2) -> [s22]
  Subsystem/3(Out3) -> [s23]
  Subsystem/4(Out4) -> [s24]
  Voltage Measurement/1 -> Product/2, Display1/1
  Current Measurement/1 -> RMS/1(In)
  Product/1 -> [P4], Scope/1
  RMS/1(RMS) -> Product/1, Display/1
  connections:
  IGBT/Diode20/LConn1 -- Current Measurement/RConn1 -- IGBT/Diode21/LConn1
  IGBT/Diode22/LConn1 -- IGBT/Diode20/RConn1 -- Conn1/RConn1
  IGBT/Diode22/RConn1 -- Voltage Measurement/LConn2 -- DC Voltage Source5/LConn1 -- IGBT/Diode23/RConn1
  IGBT/Diode23/LConn1 -- Conn2/RConn1 -- IGBT/Diode21/RConn1
  Current Measurement/LConn1 -- Voltage Measurement/LConn1 -- DC Voltage Source5/RConn1

== system SPWM/Subsystem7/RMS/RMS  ==
  In : Inport
  Enable : EnablePort
  Fourier1 : powerlib_meascontrol/Measurements/Fourier  Freq=sps.Freq  n=1  InInit=sps.Par_Init_RMS  Ts=Ts
      settings: SourceProductName=Simscape Power Systems
  Gain : Gain  Gain=1/sqrt(2)
  Terminator : Terminator
  RMS : Outport
  wires:
  Fourier1/1 -> Gain/1
  Fourier1/2 -> Terminator/1
  In/1 -> Fourier1/1
  Gain/1 -> RMS/1

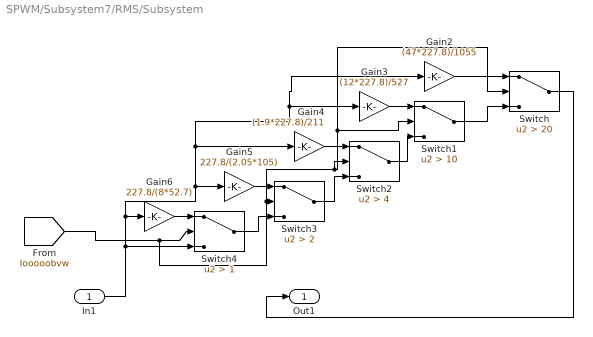
== system SPWM/Subsystem7/RMS/Subsystem ==
  In1 : Inport
  Gain2 : Gain  Gain=(47*227.8)/1055
  Gain3 : Gain  Gain=(12*227.8)/527
  Gain4 : Gain  Gain=(1.9*227.8)/211
  Gain5 : Gain  Gain=227.8/(2.05*105)
  Gain6 : Gain  Gain=227.8/(8*52.7)
  Switch : Switch  Criteria=u2 > Threshold  Threshold=20
  Switch1 : Switch  Criteria=u2 > Threshold  Threshold=10
  Switch2 : Switch  Criteria=u2 > Threshold  Threshold=4
  Switch3 : Switch  Criteria=u2 > Threshold  Threshold=2
  Switch4 : Switch  Criteria=u2 > Threshold  Threshold=1
  Out1 : Outport
  wires:
  Switch1/1 -> Switch/3
  In1/1 -> Switch4/3, Gain6/1, Gain5/1, Gain4/1, Gain3/1, Gain2/1
  [Iooooobvw] -> Switch/2, Switch1/2, Switch2/2, Switch3/2, Switch4/2
  Gain3/1 -> Switch1/1
  Switch3/1 -> Switch2/3
  Gain4/1 -> Switch2/1
  Gain5/1 -> Switch3/1
  Gain2/1 -> Switch/1
  Switch2/1 -> Switch1/3
  Switch4/1 -> Switch3/3
  Gain6/1 -> Switch4/1
  Switch/1 -> Out1/1

== system SPWM/Subsystem7/RMS/TrueRMS  ==
  In : Inport
  Enable : EnablePort
  Gain : Gain  Gain=1/13.8
  Gain1 : Gain  Gain=1400/93400
  Mean value : powerlib_meascontrol/Measurements/Mean  Freq=sps.Freq  Vinit=sps.Par_Init_TrueRMS  Ts=Ts
  Product : Product  SaturateOnIntegerOverflow=on  InputSameDT=on  OutDataTypeStr=Inherit: Same as first input
  Saturation to avoid negative sqrt : Saturate  UpperLimit=Inf  LowerLimit=0
  Sqrt : Sqrt  AlgorithmType=Newton-Raphson  SaturateOnIntegerOverflow=on
  RMS : Outport
  wires:
  Saturation to avoid negative sqrt/1 -> Sqrt/1
  Mean value/1 -> Saturation to avoid negative sqrt/1
  Product/1 -> Mean value/1
  In/1 -> Product/2, Product/1
  Sqrt/1 -> Gain/1
  Gain/1 -> Gain1/1
  Gain1/1 -> RMS/1

== system SPWM/Subsystem7/Subsystem/RMS ==
  In : Inport  SampleTime=Ts
  Constant : Constant  Value=TrueRMS
  Data Type Conversion : DataTypeConversion  OutDataTypeStr=boolean
  Logical Operator : Logic  Operator=NOT  AllPortsSameDT=off  OutDataTypeStr=boolean
  "RMS " : Subsystem
  Subsystem : Subsystem
  Switch : Switch  Criteria=u2 ~= 0  Threshold=0.5
  "TrueRMS " : Subsystem
  RMS : Outport  SampleTime=Ts
  wires:
  In/1 -> "TrueRMS "/1(In), "RMS "/1(In)
  "TrueRMS "/1(RMS) -> Switch/1
  "RMS "/1(RMS) -> Switch/3
  Constant/1 -> Data Type Conversion/1
  Data Type Conversion/1 -> Logical Operator/1, "TrueRMS "/Enable, Switch/2
  Logical Operator/1 -> "RMS "/Enable
  Switch/1 -> Subsystem/1(In1)
  Subsystem/1(Out1) -> RMS/1

== system SPWM/Subsystem7/Subsystem/Subsystem ==
  NOT : Logic  Operator=NOT  AllPortsSameDT=off  OutDataTypeStr=boolean
  NOT1 : Logic  Operator=NOT  AllPortsSameDT=off  OutDataTypeStr=boolean
  Relational Operator : RelationalOperator  OutDataTypeStr=boolean  RndMeth=Simplest
  Relational Operator1 : RelationalOperator  OutDataTypeStr=boolean  RndMeth=Simplest
  Repeating Sequence : simulink/Sources/Repeating Sequence  rep_seq_t=[0 0.0001 0.00021 0.0003 0.0004]  rep_seq_y=[0.6 0.7 0.6 0.7 0.6]
  Repeating Sequence1 : simulink/Sources/Repeating Sequence  rep_seq_t=[0 0.0001 0.00021 0.0003 0.0004]  rep_seq_y=[0.5 0.6 0.5 0.6 0.5]
  Scope : Scope  NumInputPorts=3
  Sine Wave : Sin  Amplitude=0.7  Frequency=2*pi*50  Samples=2*pi*50  SampleTime=1e-6  VectorParams1D=off
  Out1 : Outport
  Out2 : Outport  Port=2
  Out3 : Outport  Port=3
  Out4 : Outport  Port=4
  wires:
  NOT/1 -> Out2/1
  Repeating Sequence/1 -> Scope/2, Relational Operator/2
  Relational Operator/1 -> Out1/1, NOT/1
  Repeating Sequence1/1 -> Relational Operator1/2, Scope/3
  Relational Operator1/1 -> Out3/1, NOT1/1
  NOT1/1 -> Out4/1
  Sine Wave/1 -> Relational Operator1/1, Relational Operator/1, Scope/1

== system SPWM/Subsystem7/Subsystem1/RMS ==
  In : Inport  SampleTime=Ts
  Constant : Constant  Value=TrueRMS
  Data Type Conversion : DataTypeConversion  OutDataTypeStr=boolean
  Logical Operator : Logic  Operator=NOT  AllPortsSameDT=off  OutDataTypeStr=boolean
  "RMS " : Subsystem
  Subsystem : Subsystem
  Switch : Switch  Criteria=u2 ~= 0  Threshold=0.5
  "TrueRMS " : Subsystem
  RMS : Outport  SampleTime=Ts
  wires:
  In/1 -> "TrueRMS "/1(In), "RMS "/1(In)
  "TrueRMS "/1(RMS) -> Switch/1
  "RMS "/1(RMS) -> Switch/3
  Constant/1 -> Data Type Conversion/1
  Data Type Conversion/1 -> Logical Operator/1, "TrueRMS "/Enable, Switch/2
  Logical Operator/1 -> "RMS "/Enable
  Switch/1 -> Subsystem/1(In1)
  Subsystem/1(Out1) -> RMS/1

== system SPWM/Subsystem7/Subsystem1/Subsystem7 ==
  NOT12 : Logic  Operator=NOT  AllPortsSameDT=off  OutDataTypeStr=boolean
  NOT13 : Logic  Operator=NOT  AllPortsSameDT=off  OutDataTypeStr=boolean
  Relational Operator12 : RelationalOperator  OutDataTypeStr=boolean  RndMeth=Simplest
  Relational Operator13 : RelationalOperator  OutDataTypeStr=boolean  RndMeth=Simplest
  Repeating Sequence12 : simulink/Sources/Repeating Sequence  rep_seq_t=[0 0.0001 0.00021 0.0003 0.0004]  rep_seq_y=[-0.5 -0.6 -0.5 -0.6 -0.5]
  Repeating Sequence13 : simulink/Sources/Repeating Sequence  rep_seq_t=[0 0.0001 0.00021 0.0003 0.0004]  rep_seq_y=[-0.6 -0.7 -0.6 -0.7 -0.6]
  Scope : Scope  NumInputPorts=3
  Sine Wave : Sin  Amplitude=0.7  Frequency=2*pi*50  Samples=2*pi*50  SampleTime=1e-6  VectorParams1D=off
  Out1 : Outport
  Out2 : Outport  Port=2
  Out3 : Outport  Port=3
  Out4 : Outport  Port=4
  wires:
  Repeating Sequence13/1 -> Scope/3, Relational Operator13/2
  Sine Wave/1 -> Relational Operator13/1, Relational Operator12/1, Scope/1
  Repeating Sequence12/1 -> Scope/2, Relational Operator12/2
  NOT12/1 -> Out2/1
  Relational Operator13/1 -> Out3/1, NOT13/1
  Relational Operator12/1 -> Out1/1, NOT12/1
  NOT13/1 -> Out4/1

== system SPWM/Subsystem7/Subsystem2/RMS ==
  In : Inport  SampleTime=Ts
  Constant : Constant  Value=TrueRMS
  Data Type Conversion : DataTypeConversion  OutDataTypeStr=boolean
  Logical Operator : Logic  Operator=NOT  AllPortsSameDT=off  OutDataTypeStr=boolean
  "RMS " : Subsystem
  Subsystem : Subsystem
  Switch : Switch  Criteria=u2 ~= 0  Threshold=0.5
  "TrueRMS " : Subsystem
  RMS : Outport  SampleTime=Ts
  wires:
  In/1 -> "TrueRMS "/1(In), "RMS "/1(In)
  "TrueRMS "/1(RMS) -> Switch/1
  "RMS "/1(RMS) -> Switch/3
  Constant/1 -> Data Type Conversion/1
  Data Type Conversion/1 -> Logical Operator/1, "TrueRMS "/Enable, Switch/2
  Logical Operator/1 -> "RMS "/Enable
  Switch/1 -> Subsystem/1(In1)
  Subsystem/1(Out1) -> RMS/1

== system SPWM/Subsystem7/Subsystem2/Subsystem ==
  NOT2 : Logic  Operator=NOT  AllPortsSameDT=off  OutDataTypeStr=boolean
  NOT3 : Logic  Operator=NOT  AllPortsSameDT=off  OutDataTypeStr=boolean
  Relational Operator2 : RelationalOperator  OutDataTypeStr=boolean  RndMeth=Simplest
  Relational Operator3 : RelationalOperator  OutDataTypeStr=boolean  RndMeth=Simplest
  Repeating Sequence2 : simulink/Sources/Repeating Sequence  rep_seq_t=[0 0.0001 0.00021 0.0003 0.0004]  rep_seq_y=[0.4 0.5 0.4 0.5 0.4]
  Repeating Sequence3 : simulink/Sources/Repeating Sequence  rep_seq_t=[0 0.0001 0.00021 0.0003 0.0004]  rep_seq_y=[0.3 0.4 0.3 0.4 0.3]
  Scope : Scope  NumInputPorts=3
  Sine Wave : Sin  Amplitude=0.7  Frequency=2*pi*50  Samples=2*pi*50  SampleTime=1e-6  VectorParams1D=off
  Out1 : Outport
  Out2 : Outport  Port=2
  Out3 : Outport  Port=3
  Out4 : Outport  Port=4
  wires:
  Repeating Sequence3/1 -> Relational Operator3/2, Scope/3
  Repeating Sequence2/1 -> Relational Operator2/2, Scope/2
  Relational Operator2/1 -> Out1/1, NOT2/1
  NOT3/1 -> Out4/1
  Relational Operator3/1 -> Out3/1, NOT3/1
  NOT2/1 -> Out2/1
  Sine Wave/1 -> Relational Operator3/1, Relational Operator2/1, Scope/1

== system SPWM/Subsystem7/Subsystem3/RMS ==
  In : Inport  SampleTime=Ts
  Constant : Constant  Value=TrueRMS
  Data Type Conversion : DataTypeConversion  OutDataTypeStr=boolean
  Logical Operator : Logic  Operator=NOT  AllPortsSameDT=off  OutDataTypeStr=boolean
  "RMS " : Subsystem
  Subsystem : Subsystem
  Switch : Switch  Criteria=u2 ~= 0  Threshold=0.5
  "TrueRMS " : Subsystem
  RMS : Outport  SampleTime=Ts
  wires:
  In/1 -> "TrueRMS "/1(In), "RMS "/1(In)
  "TrueRMS "/1(RMS) -> Switch/1
  "RMS "/1(RMS) -> Switch/3
  Constant/1 -> Data Type Conversion/1
  Data Type Conversion/1 -> Logical Operator/1, "TrueRMS "/Enable, Switch/2
  Logical Operator/1 -> "RMS "/Enable
  Switch/1 -> Subsystem/1(In1)
  Subsystem/1(Out1) -> RMS/1

== system SPWM/Subsystem7/Subsystem3/Subsystem ==
  NOT4 : Logic  Operator=NOT  AllPortsSameDT=off  OutDataTypeStr=boolean
  NOT5 : Logic  Operator=NOT  AllPortsSameDT=off  OutDataTypeStr=boolean
  Relational Operator4 : RelationalOperator  OutDataTypeStr=boolean  RndMeth=Simplest
  Relational Operator5 : RelationalOperator  OutDataTypeStr=boolean  RndMeth=Simplest
  Repeating Sequence4 : simulink/Sources/Repeating Sequence  rep_seq_t=[0 0.0001 0.00021 0.0003 0.0004]  rep_seq_y=[0.2 0.3 0.2 0.3 0.2]
  Repeating Sequence5 : simulink/Sources/Repeating Sequence  rep_seq_t=[0 0.0001 0.00021 0.0003 0.0004]  rep_seq_y=[0.1 0.2 0.1 0.2 0.1]
  Scope : Scope  NumInputPorts=3
  Sine Wave : Sin  Amplitude=0.7  Frequency=2*pi*50  Samples=2*pi*50  SampleTime=1e-6  VectorParams1D=off
  Out1 : Outport
  Out2 : Outport  Port=2
  Out3 : Outport  Port=3
  Out4 : Outport  Port=4
  wires:
  NOT4/1 -> Out2/1
  Repeating Sequence4/1 -> Relational Operator4/2, Scope/2
  NOT5/1 -> Out4/1
  Relational Operator4/1 -> Out1/1, NOT4/1
  Relational Operator5/1 -> Out3/1, NOT5/1
  Repeating Sequence5/1 -> Relational Operator5/2, Scope/3
  Sine Wave/1 -> Relational Operator5/1, Relational Operator4/1, Scope/1

== system SPWM/Subsystem7/Subsystem4/RMS ==
  In : Inport  SampleTime=Ts
  Constant : Constant  Value=TrueRMS
  Data Type Conversion : DataTypeConversion  OutDataTypeStr=boolean
  Logical Operator : Logic  Operator=NOT  AllPortsSameDT=off  OutDataTypeStr=boolean
  "RMS " : Subsystem
  Subsystem : Subsystem
  Switch : Switch  Criteria=u2 ~= 0  Threshold=0.5
  "TrueRMS " : Subsystem
  RMS : Outport  SampleTime=Ts
  wires:
  In/1 -> "TrueRMS "/1(In), "RMS "/1(In)
  "TrueRMS "/1(RMS) -> Switch/1
  "RMS "/1(RMS) -> Switch/3
  Constant/1 -> Data Type Conversion/1
  Data Type Conversion/1 -> Logical Operator/1, "TrueRMS "/Enable, Switch/2
  Logical Operator/1 -> "RMS "/Enable
  Switch/1 -> Subsystem/1(In1)
  Subsystem/1(Out1) -> RMS/1

== system SPWM/Subsystem7/Subsystem4/Subsystem ==
  NOT6 : Logic  Operator=NOT  AllPortsSameDT=off  OutDataTypeStr=boolean
  NOT7 : Logic  Operator=NOT  AllPortsSameDT=off  OutDataTypeStr=boolean
  Relational Operator6 : RelationalOperator  OutDataTypeStr=boolean  RndMeth=Simplest
  Relational Operator7 : RelationalOperator  OutDataTypeStr=boolean  RndMeth=Simplest
  Repeating Sequence6 : simulink/Sources/Repeating Sequence  rep_seq_t=[0 0.0001 0.00021 0.0003 0.0004]  rep_seq_y=[0 0.1 0 0.1 0 ]
  Repeating Sequence7 : simulink/Sources/Repeating Sequence  rep_seq_t=[0 0.0001 0.00021 0.0003 0.0004]  rep_seq_y=[-0.1 0 -0.1 0 -0.1]
  Scope : Scope  NumInputPorts=3
  Sine Wave : Sin  Amplitude=0.7  Frequency=2*pi*50  Samples=2*pi*50  SampleTime=1e-6  VectorParams1D=off
  Out1 : Outport
  Out2 : Outport  Port=2
  Out3 : Outport  Port=3
  Out4 : Outport  Port=4
  wires:
  Repeating Sequence6/1 -> Scope/2, Relational Operator6/2
  NOT6/1 -> Out2/1
  Relational Operator7/1 -> Out3/1, NOT7/1
  Repeating Sequence7/1 -> Scope/3, Relational Operator7/2
  NOT7/1 -> Out4/1
  Relational Operator6/1 -> Out1/1, NOT6/1
  Sine Wave/1 -> Scope/1, Relational Operator7/1, Relational Operator6/1

== system SPWM/Subsystem7/Subsystem5/RMS ==
  In : Inport  SampleTime=Ts
  Constant : Constant  Value=TrueRMS
  Data Type Conversion : DataTypeConversion  OutDataTypeStr=boolean
  Logical Operator : Logic  Operator=NOT  AllPortsSameDT=off  OutDataTypeStr=boolean
  "RMS " : Subsystem
  Subsystem : Subsystem
  Switch : Switch  Criteria=u2 ~= 0  Threshold=0.5
  "TrueRMS " : Subsystem
  RMS : Outport  SampleTime=Ts
  wires:
  In/1 -> "TrueRMS "/1(In), "RMS "/1(In)
  "TrueRMS "/1(RMS) -> Switch/1
  "RMS "/1(RMS) -> Switch/3
  Constant/1 -> Data Type Conversion/1
  Data Type Conversion/1 -> Logical Operator/1, "TrueRMS "/Enable, Switch/2
  Logical Operator/1 -> "RMS "/Enable
  Switch/1 -> Subsystem/1(In1)
  Subsystem/1(Out1) -> RMS/1

== system SPWM/Subsystem7/Subsystem5/Subsystem ==
  NOT8 : Logic  Operator=NOT  AllPortsSameDT=off  OutDataTypeStr=boolean
  NOT9 : Logic  Operator=NOT  AllPortsSameDT=off  OutDataTypeStr=boolean
  Relational Operator8 : RelationalOperator  OutDataTypeStr=boolean  RndMeth=Simplest
  Relational Operator9 : RelationalOperator  OutDataTypeStr=boolean  RndMeth=Simplest
  Repeating Sequence8 : simulink/Sources/Repeating Sequence  rep_seq_t=[0 0.0001 0.00021 0.0003 0.0004]  rep_seq_y=[-0.2 -0.1 -0.2 -0.1 -0.2]
  Repeating Sequence9 : simulink/Sources/Repeating Sequence  rep_seq_t=[0 0.0001 0.00021 0.0003 0.0004]  rep_seq_y=[-0.3 -0.2 -0.3 -0.2 -0.3]
  Scope : Scope  NumInputPorts=3
  Sine Wave : Sin  Amplitude=0.7  Frequency=2*pi*50  Samples=2*pi*50  SampleTime=1e-6  VectorParams1D=off
  Out1 : Outport
  Out2 : Outport  Port=2
  Out3 : Outport  Port=3
  Out4 : Outport  Port=4
  wires:
  Repeating Sequence8/1 -> Scope/2, Relational Operator8/2
  Relational Operator9/1 -> Out3/1, NOT9/1
  Relational Operator8/1 -> Out1/1, NOT8/1
  NOT9/1 -> Out4/1
  Repeating Sequence9/1 -> Relational Operator9/2
  NOT8/1 -> Out2/1
  Sine Wave/1 -> Relational Operator9/1, Relational Operator8/1, Scope/3, Scope/1

== system SPWM/Subsystem7/Subsystem6/RMS ==
  In : Inport  SampleTime=Ts
  Constant : Constant  Value=TrueRMS
  Data Type Conversion : DataTypeConversion  OutDataTypeStr=boolean
  Logical Operator : Logic  Operator=NOT  AllPortsSameDT=off  OutDataTypeStr=boolean
  "RMS " : Subsystem
  Subsystem : Subsystem
  Switch : Switch  Criteria=u2 ~= 0  Threshold=0.5
  "TrueRMS " : Subsystem
  RMS : Outport  SampleTime=Ts
  wires:
  In/1 -> "TrueRMS "/1(In), "RMS "/1(In)
  "TrueRMS "/1(RMS) -> Switch/1
  "RMS "/1(RMS) -> Switch/3
  Constant/1 -> Data Type Conversion/1
  Data Type Conversion/1 -> Logical Operator/1, "TrueRMS "/Enable, Switch/2
  Logical Operator/1 -> "RMS "/Enable
  Switch/1 -> Subsystem/1(In1)
  Subsystem/1(Out1) -> RMS/1

== system SPWM/Subsystem7/Subsystem6/Subsystem ==
  NOT10 : Logic  Operator=NOT  AllPortsSameDT=off  OutDataTypeStr=boolean
  NOT11 : Logic  Operator=NOT  AllPortsSameDT=off  OutDataTypeStr=boolean
  Relational Operator10 : RelationalOperator  OutDataTypeStr=boolean  RndMeth=Simplest
  Relational Operator11 : RelationalOperator  OutDataTypeStr=boolean  RndMeth=Simplest
  Repeating Sequence10 : simulink/Sources/Repeating Sequence  rep_seq_t=[0 0.0001 0.00021 0.0003 0.0004]  rep_seq_y=[-0.3 -0.4 -0.3 -0.4 -0.3]
  Repeating Sequence11 : simulink/Sources/Repeating Sequence  rep_seq_t=[0 0.0001 0.00021 0.0003 0.0004]  rep_seq_y=[-0.4 -0.5 -0.4 -0.5 -0.4]
  Scope : Scope  NumInputPorts=3
  Sine Wave : Sin  Amplitude=0.7  Frequency=2*pi*50  Samples=2*pi*50  SampleTime=1e-6  VectorParams1D=off
  Out1 : Outport
  Out2 : Outport  Port=2
  Out3 : Outport  Port=3
  Out4 : Outport  Port=4
  wires:
  Relational Operator11/1 -> Out3/1, NOT11/1
  Relational Operator10/1 -> Out1/1, NOT10/1
  Repeating Sequence11/1 -> Scope/3, Relational Operator11/2
  NOT10/1 -> Out2/1
  Repeating Sequence10/1 -> Relational Operator10/2, Scope/2
  NOT11/1 -> Out4/1
  Sine Wave/1 -> Relational Operator11/1, Relational Operator10/1, Scope/1

== system SPWM/Subsystem7/Subsystem/RMS/RMS  ==
  In : Inport
  Enable : EnablePort
  Fourier1 : powerlib_meascontrol/Measurements/Fourier  Freq=sps.Freq  n=1  InInit=sps.Par_Init_RMS  Ts=Ts
      settings: SourceProductName=Simscape Power Systems
  Gain : Gain  Gain=1/sqrt(2)
  Terminator : Terminator
  RMS : Outport
  wires:
  Fourier1/1 -> Gain/1
  Fourier1/2 -> Terminator/1
  In/1 -> Fourier1/1
  Gain/1 -> RMS/1

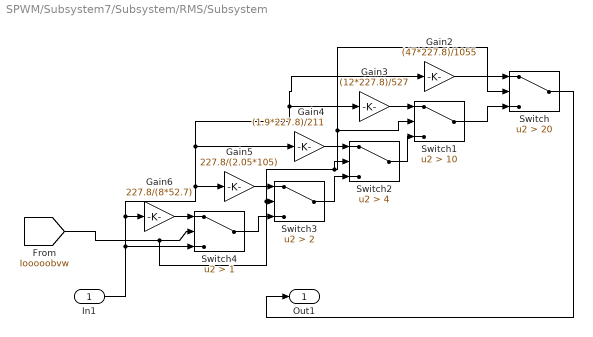
== system SPWM/Subsystem7/Subsystem/RMS/Subsystem ==
  In1 : Inport
  Gain2 : Gain  Gain=(47*227.8)/1055
  Gain3 : Gain  Gain=(12*227.8)/527
  Gain4 : Gain  Gain=(1.9*227.8)/211
  Gain5 : Gain  Gain=227.8/(2.05*105)
  Gain6 : Gain  Gain=227.8/(8*52.7)
  Switch : Switch  Criteria=u2 > Threshold  Threshold=20
  Switch1 : Switch  Criteria=u2 > Threshold  Threshold=10
  Switch2 : Switch  Criteria=u2 > Threshold  Threshold=4
  Switch3 : Switch  Criteria=u2 > Threshold  Threshold=2
  Switch4 : Switch  Criteria=u2 > Threshold  Threshold=1
  Out1 : Outport
  wires:
  Switch1/1 -> Switch/3
  In1/1 -> Switch4/3, Gain6/1, Gain5/1, Gain4/1, Gain3/1, Gain2/1
  [Iooooobvw] -> Switch/2, Switch1/2, Switch2/2, Switch3/2, Switch4/2
  Gain3/1 -> Switch1/1
  Switch3/1 -> Switch2/3
  Gain4/1 -> Switch2/1
  Gain5/1 -> Switch3/1
  Gain2/1 -> Switch/1
  Switch2/1 -> Switch1/3
  Switch4/1 -> Switch3/3
  Gain6/1 -> Switch4/1
  Switch/1 -> Out1/1

== system SPWM/Subsystem7/Subsystem/RMS/TrueRMS  ==
  In : Inport
  Enable : EnablePort
  Gain : Gain  Gain=1/13.8
  Gain1 : Gain  Gain=1400/93400
  Mean value : powerlib_meascontrol/Measurements/Mean  Freq=sps.Freq  Vinit=sps.Par_Init_TrueRMS  Ts=Ts
  Product : Product  SaturateOnIntegerOverflow=on  InputSameDT=on  OutDataTypeStr=Inherit: Same as first input
  Saturation to avoid negative sqrt : Saturate  UpperLimit=Inf  LowerLimit=0
  Sqrt : Sqrt  AlgorithmType=Newton-Raphson  SaturateOnIntegerOverflow=on
  RMS : Outport
  wires:
  Saturation to avoid negative sqrt/1 -> Sqrt/1
  Mean value/1 -> Saturation to avoid negative sqrt/1
  Product/1 -> Mean value/1
  In/1 -> Product/2, Product/1
  Sqrt/1 -> Gain/1
  Gain/1 -> Gain1/1
  Gain1/1 -> RMS/1

== system SPWM/Subsystem7/Subsystem1/RMS/RMS  ==
  In : Inport
  Enable : EnablePort
  Fourier1 : powerlib_meascontrol/Measurements/Fourier  Freq=sps.Freq  n=1  InInit=sps.Par_Init_RMS  Ts=Ts
      settings: SourceProductName=Simscape Power Systems
  Gain : Gain  Gain=1/sqrt(2)
  Terminator : Terminator
  RMS : Outport
  wires:
  Fourier1/1 -> Gain/1
  Fourier1/2 -> Terminator/1
  In/1 -> Fourier1/1
  Gain/1 -> RMS/1
